simulink model "midterm_q5"  (R2022b)
settings: Solver=VariableStepAuto  StartTime=0.0  StopTime=10.0  RelTol=1e-3
settings Model: Creator=gaura  LastModifiedBy=gaura

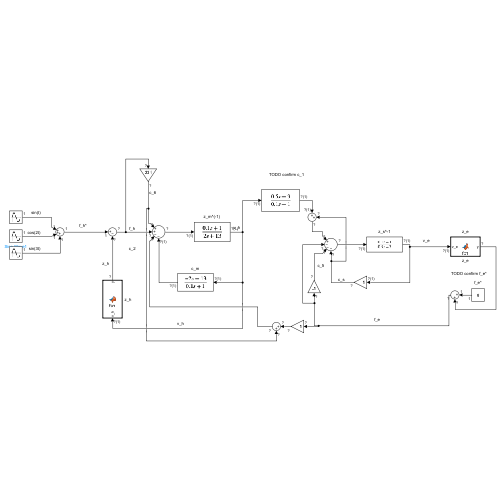
[thumbnail: Simulink's stored preview of the top-level diagram]
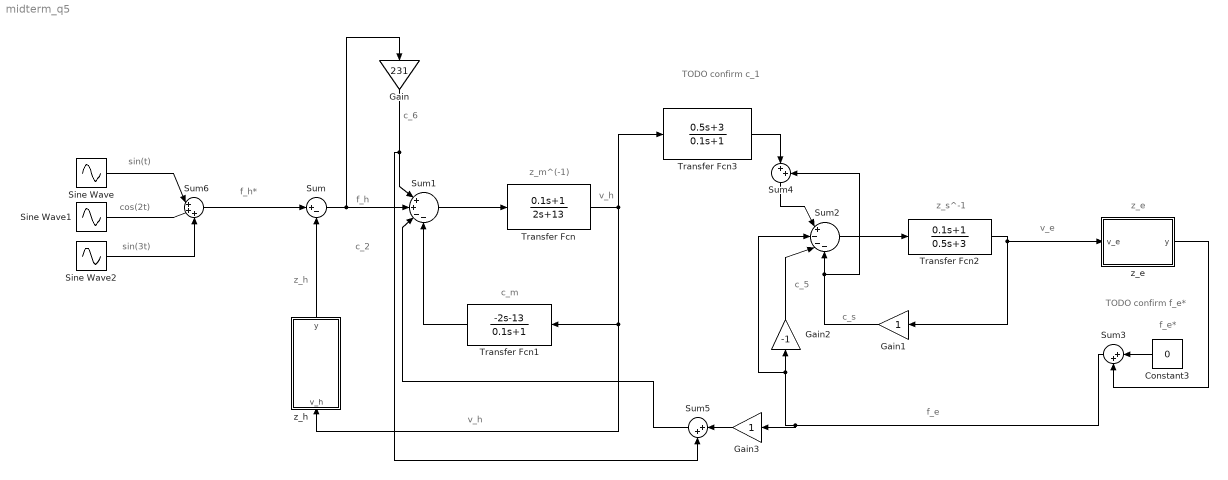
== system midterm_q5 ==
  note: sin(3t)
  note: cos(2t)
  note: sin(t)
  note: f_e
  note: TODO confirm f_e*
  note: f_e*
  note: z_e
  note: v_e
  note: z_s^-1
  note: c_5
  note: TODO confirm c_1
  note: c_s
  note: c_m
  note: v_h
  note: z_m^(-1)
  note: c_6
  note: c_2
  note: f_h
  note: z_h
  note: f_h*
  note: v_h
  Constant3 : Constant  Value=0
  Gain : Gain  Gain=231
  Gain1 : Gain
  Gain2 : Gain  Gain=-1
  Gain3 : Gain
  Sine Wave : Sin  SampleTime=0
  Sine Wave1 : Sin  Frequency=2  Phase=pi/2  SampleTime=0
  Sine Wave2 : Sin  SampleTime=0
  Sum : Sum  Inputs=|+-
  Sum1 : Sum  Inputs=|++--
  Sum2 : Sum  Inputs=|+---
  Sum3 : Sum  Inputs=|++
  Sum4 : Sum  Inputs=|++
  Sum5 : Sum  Inputs=|++
  Sum6 : Sum  Inputs=|+++
  Transfer Fcn : TransferFcn  Numerator=[0.1 1]  Denominator=[2 13]
  Transfer Fcn1 : TransferFcn  Numerator=[-2 -13]  Denominator=[0.1 1]
  Transfer Fcn2 : TransferFcn  Numerator=[0.1 1]  Denominator=[0.5 3]
  Transfer Fcn3 : TransferFcn  Numerator=[0.5 3]  Denominator=[0.1 1]
  z_e : MATLAB Function  TreatAsAtomicUnit=on
  z_h : MATLAB Function  TreatAsAtomicUnit=on
  wires:
  Sum6/1 -> Sum/1
  z_h/1(y) -> Sum/2
  Sum/1 -> Gain/1, Sum1/2
  Gain/1 -> Sum1/1, Sum5/2
  Sum1/1 -> Transfer Fcn/1
  Gain1/1 -> Sum4/2, Sum2/4
  Transfer Fcn1/1 -> Sum1/4
  Gain2/1 -> Sum2/3
  Transfer Fcn2/1 -> Gain1/1, z_e/1(v_e)
  Sum2/1 -> Transfer Fcn2/1
  z_e/1(y) -> Sum3/2
  Constant3/1 -> Sum3/1
  Sum3/1 -> Gain3/1, Sum2/2, Gain2/1
  Transfer Fcn/1 -> Transfer Fcn3/1, z_h/1(v_h), Transfer Fcn1/1
  Transfer Fcn3/1 -> Sum4/1
  Sum4/1 -> Sum2/1
  Gain3/1 -> Sum5/1
  Sum5/1 -> Sum1/3
  Sine Wave/1 -> Sum6/1
  Sine Wave1/1 -> Sum6/2
  Sine Wave2/1 -> Sum6/3

== matlab function midterm_q5/z_e ==
  data: v_e input; y output
function y = fcn(v_e)

mass = 0.1;
damp_coeff = 0.5;

acc_e = diff(v_e);

y = mass*acc_e + damp_coeff*v_e;

== matlab function midterm_q5/z_h ==
  data: v_h input; y output
function y = fcn(v_h)

mass = 2;
damp_coeff = 9;

acc_h = diff(v_h);

y = mass*acc_h + damp_coeff*v_h;
